simulink model "AUDIO_EQUILIZER"  (R2025b)
settings: Solver=VariableStepAuto  StartTime=0.0  StopTime=10.0  RelTol=1e-3
libraries: fl_lib x32, nesl_utility x10, ee_lib x4
settings Model: Creator=kalas  LastModifiedBy=kalas

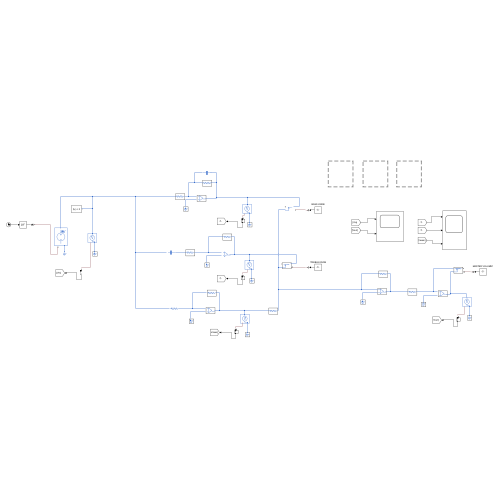
[thumbnail: Simulink's stored preview of the top-level diagram]
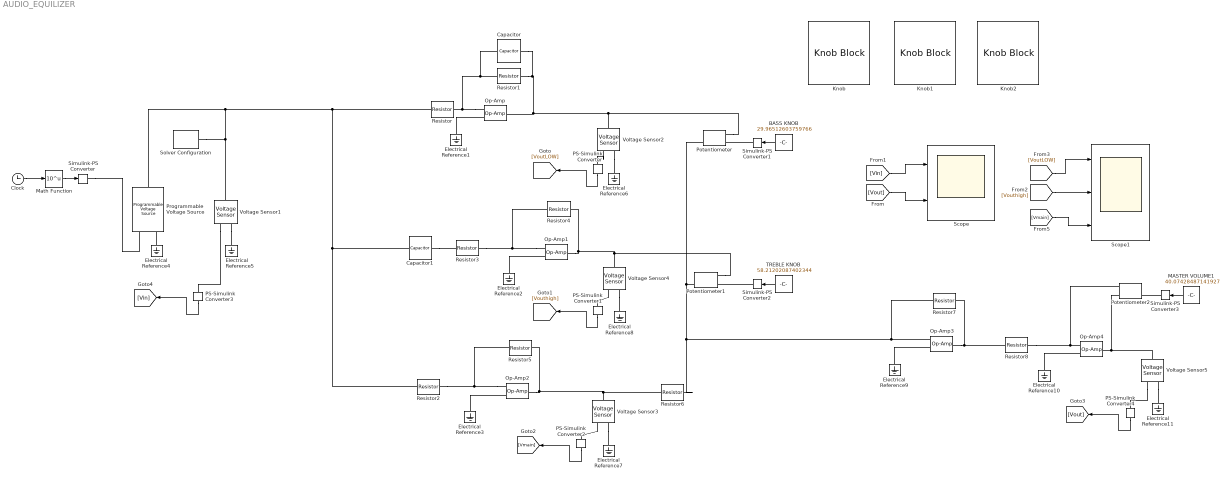
== system AUDIO_EQUILIZER ==
  BASS KNOB : Constant  Value=29.96512603759766
  Capacitor : fl_lib/Electrical/Electrical Elements/Capacitor  c=6.366 uF  r=1e-6 Ohm  g=0 1/Ohm  i_specify=off  i_priority=None  i=0 A  i_nominal_specify=off  i_nominal_value=1  i_nominal_unit=A  v_specify=off  v_priority=None  v=0 V  v_nominal_specify=off  v_nominal_value=1  v_nominal_unit=V  vc_specify=off  vc_priority=High  vc=0 V  vc_nominal_specify=off  vc_nominal_value=1  vc_nominal_unit=V
  Capacitor1 : fl_lib/Electrical/Electrical Elements/Capacitor  c=0.3979 uF  r=1e-6 Ohm  g=0 1/Ohm  i_specify=off  i_priority=None  i=0 A  i_nominal_specify=off  i_nominal_value=1  i_nominal_unit=A  v_specify=off  v_priority=None  v=0 V  v_nominal_specify=off  v_nominal_value=1  v_nominal_unit=V  vc_specify=off  vc_priority=High  vc=0 V  vc_nominal_specify=off  vc_nominal_value=1  vc_nominal_unit=V
  Clock : Clock
  Electrical Reference{1..11} (11 alike) : fl_lib/Electrical/Electrical Elements/Electrical Reference
  Knob : KnobBlock
  Knob1 : KnobBlock
  Knob2 : KnobBlock
  MASTER VOLUME1 : Constant  Value=40.07428487141927
  Math Function : Math  Operator=10^u
  Op-Amp{,1..4} (5 alike) : fl_lib/Electrical/Electrical Elements/Op-Amp  outI_specify=off  outI_priority=None  outI=0 A  outI_nominal_specify=off  outI_nominal_value=1  outI_nominal_unit=A
  PS-Simulink Converter{,1..4} (5 alike) : nesl_utility/PS-Simulink Converter  PhysicalDomain=network_engine_domain  SubClassName=ps_output  LeftPortType=input  RightPortType=output  PseudoPeriodic=off  Frequencies=[]  VectorFormat=inherit  Unit=inherit  AffineConversion=off
  Potentiometer : ee_lib/Passive/Potentiometer  nPorts=ee.enum.passive.potentiometer.nPorts.Three  R0=1000 Ohm  Rw=1 Ohm  xmin=0  xmax=1  minResistance=1 Ohm  maxResistance=999 Ohm  xmin2port=0  xmax2port=1  Taper=ee.enum.passive.potentiometer.linOrLog.lin  Rcenter=200 Ohm  Gradient=ee.enum.passive.potentiometer.gradient.higherR
      settings: InternalSimscapePortConfiguration="{\"Bottom\":[],\"Left\":[{\"id\":\"pinL\",\"label\":\"L\",\"type\":\"foundation.electrical.electrical\"},{\"id\":\"W\",\"label\":\"W\",\"type\":\"foundation.electrical.electrical\"}],\"Right\":[{\"id\":\"pinR\",\"label\":\"R\",\"type\":\"foundation.electrical.electrical\"},{\"id\":\"x\",\"label\":\"x\",\"type\":\"input\"}],\"Top\":[]}"
  Potentiometer1 : ee_lib/Passive/Potentiometer  nPorts=ee.enum.passive.potentiometer.nPorts.Three  R0=1000 Ohm  Rw=1 Ohm  xmin=0  xmax=1  minResistance=1 Ohm  maxResistance=999 Ohm  xmin2port=0  xmax2port=1  Taper=ee.enum.passive.potentiometer.linOrLog.lin  Rcenter=200 Ohm  Gradient=ee.enum.passive.potentiometer.gradient.higherR
      settings: InternalSimscapePortConfiguration="{\"Bottom\":[],\"Left\":[{\"id\":\"pinL\",\"label\":\"L\",\"type\":\"foundation.electrical.electrical\"},{\"id\":\"W\",\"label\":\"W\",\"type\":\"foundation.electrical.electrical\"}],\"Right\":[{\"id\":\"pinR\",\"label\":\"R\",\"type\":\"foundation.electrical.electrical\"},{\"id\":\"x\",\"label\":\"x\",\"type\":\"input\"}],\"Top\":[]}"
  Potentiometer2 : ee_lib/Passive/Potentiometer  nPorts=ee.enum.passive.potentiometer.nPorts.Three  R0=1000 Ohm  Rw=1 Ohm  xmin=0  xmax=1  minResistance=1 Ohm  maxResistance=999 Ohm  xmin2port=0  xmax2port=1  Taper=ee.enum.passive.potentiometer.linOrLog.lin  Rcenter=200 Ohm  Gradient=ee.enum.passive.potentiometer.gradient.higherR
      settings: InternalSimscapePortConfiguration="{\"Bottom\":[],\"Left\":[{\"id\":\"pinL\",\"label\":\"L\",\"type\":\"foundation.electrical.electrical\"},{\"id\":\"W\",\"label\":\"W\",\"type\":\"foundation.electrical.electrical\"}],\"Right\":[{\"id\":\"pinR\",\"label\":\"R\",\"type\":\"foundation.electrical.electrical\"},{\"id\":\"x\",\"label\":\"x\",\"type\":\"input\"}],\"Top\":[]}"
  Programmable Voltage Source : ee_lib/Sources/Programmable Voltage Source  magnitude_type=ee.enum.timechanging.constant  ac_magnitude=10 V  magn_ramp=1 V/s  magn_step=1 V  magn_modu_magn=1 V  magn_modu_freq=1 Hz  magn_t1=1 s  magn_t2=2 s  frequency_type=ee.enum.timechanging.external  ac_frequency=60 Hz  freq_ramp=1 Hz/s  freq_step=1 Hz  freq_modu_magn=1 Hz  freq_modu_freq=1 Hz  freq_t1=1 s  freq_t2=2 s  phase_type=ee.enum.timechanging.constant  ac_shift=0 deg  phase_ramp=1 deg/s  phase_step=1 deg  phase_modu_magn=1 deg  phase_modu_freq=1 Hz  phase_t1=1 s  phase_t2=2 s  dc_type=ee.enum.timechanging.constant  dc_voltage=0 V  dc_ramp=1 V/s  dc_step=1 V  dc_modu_magn=1 V  dc_modu_freq=1 Hz  dc_t1=1 s  dc_t2=2 s  harmonic_option=0  harmonic_orders=[5, 7, 11, 13]  harmonic_ratios=[.1, .1, .1, .1]  harmonic_shifts=[0, 0, 0, 0] deg  harmonic_t1=-inf s  harmonic_t2=inf s  noise_mode=0  PSD=0 V^2/Hz  repeatability=1  auto_seed=0  user_seed=0  sample_time=1e-3 s  i_specify=off  i_priority=None  i=0 A  i_nominal_specify=off  i_nominal_value=1  i_nominal_unit=A  v_specify=off  v_priority=None  v=0 V  v_nominal_specify=off  v_nominal_value=1  v_nominal_unit=V
      settings: InternalSimscapePortConfiguration="{\"Bottom\":[],\"Left\":[{\"id\":\"p\",\"label\":\"+\",\"type\":\"foundation.electrical.electrical\"}],\"Right\":[{\"id\":\"ext_freq\",\"label\":\"F\",\"type\":\"input\"},{\"id\":\"n\",\"label\":\"-\",\"type\":\"foundation.electrical.electrical\"}],\"Top\":[]}"
  Resistor{,2..8} (8 alike) : fl_lib/Electrical/Electrical Elements/Resistor  R=100 Ohm  i_specify=off  i_priority=None  i=0 A  i_nominal_specify=off  i_nominal_value=1  i_nominal_unit=A  v_specify=off  v_priority=None  v=0 V  v_nominal_specify=off  v_nominal_value=1  v_nominal_unit=V
  Resistor1 : fl_lib/Electrical/Electrical Elements/Resistor  R=50 Ohm  i_specify=off  i_priority=None  i=0 A  i_nominal_specify=off  i_nominal_value=1  i_nominal_unit=A  v_specify=off  v_priority=None  v=0 V  v_nominal_specify=off  v_nominal_value=1  v_nominal_unit=V
  Scope : Scope  NumInputPorts=2
      settings: ActiveDisplayYMinimum=-21.363071636211536  ActiveDisplayYMaximum=17.672725613110412
  Scope1 : Scope  NumInputPorts=3
      settings: ActiveDisplayYMinimum=-21.363071636211536  ActiveDisplayYMaximum=17.672725613110412
  Simulink-PS Converter{,1..3} (4 alike) : nesl_utility/Simulink-PS Converter  PhysicalDomain=network_engine_domain  SubClassName=ps_input  LeftPortType=input  RightPortType=output  PseudoPeriodic=off  Frequencies=[]  NoiseDistribution=none  NoiseParameters=[]  Unit=1  AffineConversion=off  FilteringAndDerivatives=provide  SimscapeFilterOrder=1  InputFilterTimeConstant=0.001  UdotUserProvided=0
  Solver Configuration : nesl_utility/Solver Configuration  PhysicalDomain=network_engine_domain  SubClassName=solver  LeftPortType=input  RightPortType=generic  Tones=[]  Harmonics=[]  SimulateNoise=off  Profile=off  UseLocalSampling=off  EnableSwitchedLinearOptims=on  FrequencyDomain=off  UseCCode=off  RelTol=0.001  AbsTol=0.001  MinStep=1e-09  ToWorkspace=off  RevertToSquareIcSolve=off  NumHomotopyIterations=100  PhasorMode=off  PhasorModeNumHarmonics=1  ConsistencySolver=NEWTON_XTOL_AFTER_FTOL  IndexReductionMethod=DerivativeReplacement  DoDC=off  ResidualTolerance=1e-09  ConsistencyTolSource=GLOBAL  ConsistencyAbsTol=0.001  ConsistencyRelTol=0.001  ConsistencyTolFactor=0.001  UseLocalSolver=off  LocalSolverChoice=NE_BACKWARD_EULER_ADVANCER  ResolveIndetEquations=on  FunctionEvalNumThread=1  LocalSolverSampleTime=0.001  DoFixedCost=off  MaxNonlinIter=3  MaxModeIter=2  ComputeImpulses=off  ImpulseIterations=2  LinearAlgebra=auto  LinearAlgebraNumThread=0  EquationFormulation=NE_TIME_EF  DelaysMemoryBudget=1024  AutomaticFiltering=on  FilteringTimeConstant=0.001  PartitionStorageMethod=AS_NEEDED  PartitionMemoryBudget=1024  PartitionMethod=ROBUST  MultibodyUseLocalSolver=off  MultibodyLocalSolverChoice=ODE1  MultibodyLocalSolverSampleTime=0.001
  TREBLE KNOB : Constant  Value=58.21202087402344
  Voltage Sensor{1..5} (5 alike) : fl_lib/Electrical/Electrical Sensors/Voltage Sensor
  wires:
  Math Function/1 -> Simulink-PS Converter/1
  Clock/1 -> Math Function/1
  BASS KNOB/1 -> Simulink-PS Converter1/1
  TREBLE KNOB/1 -> Simulink-PS Converter2/1
  MASTER VOLUME1/1 -> Simulink-PS Converter3/1
  PS-Simulink Converter/1 -> [VoutLOW]
  PS-Simulink Converter1/1 -> [Vouthigh]
  PS-Simulink Converter2/1 -> [Vmain]
  PS-Simulink Converter3/1 -> [Vin]
  PS-Simulink Converter4/1 -> [Vout]
  [Vout] -> Scope/2
  [Vin] -> Scope/1
  [Vouthigh] -> Scope1/2
  [VoutLOW] -> Scope1/1
  [Vmain] -> Scope1/3
  connections:
  Capacitor/RConn1 -- Resistor1/RConn1 -- Potentiometer/RConn1 -- Voltage Sensor2/LConn1 -- Op-Amp/RConn1
  Op-Amp/LConn2 -- Resistor1/LConn1 -- Capacitor/LConn1 -- Resistor/RConn1
  Op-Amp/LConn1 -- Electrical Reference1/LConn1
  Op-Amp1/LConn1 -- Electrical Reference2/LConn1
  Op-Amp1/LConn2 -- Resistor3/RConn1 -- Resistor4/LConn1
  Capacitor1/RConn1 -- Resistor3/LConn1
  Op-Amp1/RConn1 -- Potentiometer1/RConn1 -- Voltage Sensor4/LConn1 -- Resistor4/RConn1
  Op-Amp2/LConn2 -- Resistor2/RConn1 -- Resistor5/LConn1
  Op-Amp2/RConn1 -- Resistor6/LConn1 -- Voltage Sensor3/LConn1 -- Resistor5/RConn1
  Op-Amp2/LConn1 -- Electrical Reference3/LConn1
  Simulink-PS Converter/RConn1 -- Programmable Voltage Source/RConn1
  Electrical Reference4/LConn1 -- Programmable Voltage Source/RConn2
  Voltage Sensor1/RConn2 -- Electrical Reference5/LConn1
  Programmable Voltage Source/LConn1 -- Solver Configuration/RConn1 -- Voltage Sensor1/LConn1 -- Resistor2/LConn1 -- Capacitor1/LConn1 -- Resistor/LConn1
  Voltage Sensor2/RConn2 -- Electrical Reference6/LConn1
  Voltage Sensor3/RConn2 -- Electrical Reference7/LConn1
  Voltage Sensor4/RConn2 -- Electrical Reference8/LConn1
  Resistor6/RConn1 -- Resistor7/LConn1 -- Op-Amp3/LConn2 -- Potentiometer/LConn2 -- Potentiometer1/LConn2
  Op-Amp3/RConn1 -- Resistor8/LConn1 -- Resistor7/RConn1
  Op-Amp3/LConn1 -- Electrical Reference9/LConn1
  Op-Amp4/LConn1 -- Electrical Reference10/LConn1
  Resistor8/RConn1 -- Potentiometer2/LConn1 -- Op-Amp4/LConn2
  Op-Amp4/RConn1 -- Voltage Sensor5/LConn1 -- Potentiometer2/LConn2
  Voltage Sensor5/RConn2 -- Electrical Reference11/LConn1
  Simulink-PS Converter1/RConn1 -- Potentiometer/RConn2
  Simulink-PS Converter2/RConn1 -- Potentiometer1/RConn2
  Simulink-PS Converter3/RConn1 -- Potentiometer2/RConn2
  Voltage Sensor2/RConn1 -- PS-Simulink Converter/LConn1
  Voltage Sensor4/RConn1 -- PS-Simulink Converter1/LConn1
  Voltage Sensor3/RConn1 -- PS-Simulink Converter2/LConn1
  Voltage Sensor1/RConn1 -- PS-Simulink Converter3/LConn1
  Voltage Sensor5/RConn1 -- PS-Simulink Converter4/LConn1
